simulink model "Neurofeedback_GetConnectivy_Validation"  (R2021b)
settings: Solver=VariableStepAuto  StartTime=0.0  StopTime=90  RelTol=1e-3
libraries: simrfV2util1 x6, simulink x3, simrfV2elements x2
settings Model: Creator=mariodelossantos  LastModifiedBy=mariodelossantos

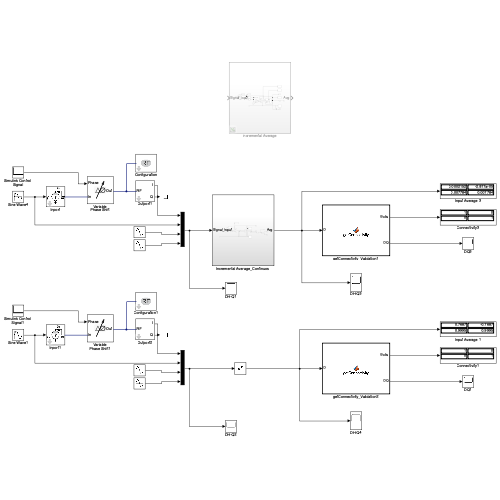
[thumbnail: Simulink's stored preview of the top-level diagram]
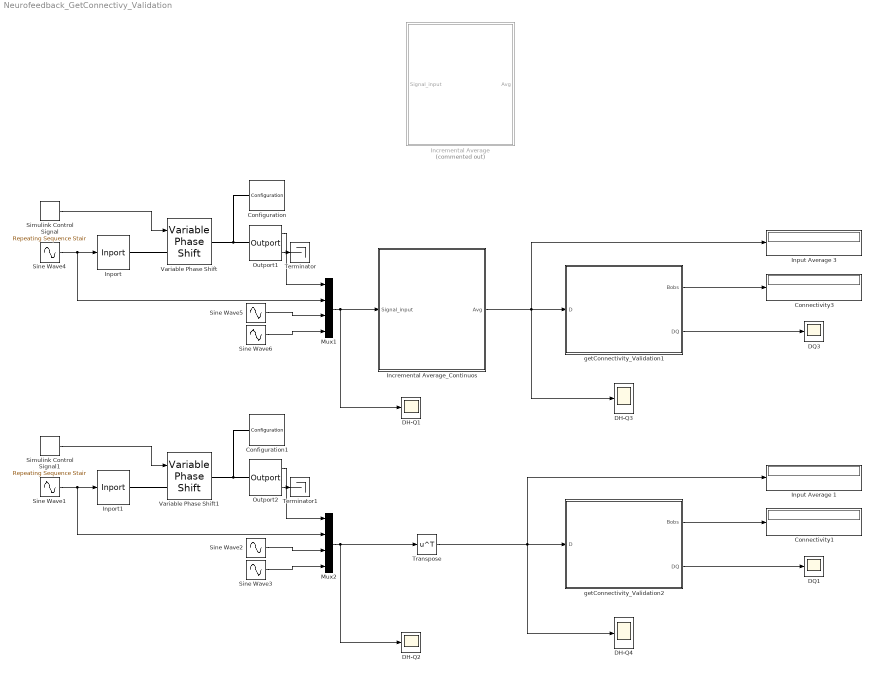
== system Neurofeedback_GetConnectivy_Validation ==
  Configuration : simrfV2util1/Configuration  AutoFreq=on  Tones=[1] GHz  Harmonics=[7]  NormalizeCarrierPower=on  SolverType=Auto  UseCCode=on  StepSize=1e-3/8 s  AddNoise=on  defaultRNG=on  Seed=0  Temperature=290.0 K  SolverDelFlag=0  AbsTol=1e-6  RelTol=1e-3  MaxIter=10  ErrorEstimationType=2-norm over all variables  EnableInterpFilter=off  HiddenFIRfilterControllerParam=on  SmallSignalApprox=off  AllSimFreqs=on  SimFreqs=[] Hz  SimFreqsInternal=[]  SamplesPerFrame=1
      settings: SourceProductBaseCode=RB
  Configuration1 : simrfV2util1/Configuration  AutoFreq=on  Tones=[1] GHz  Harmonics=[7]  NormalizeCarrierPower=on  SolverType=Auto  UseCCode=on  StepSize=1e-3/8 s  AddNoise=on  defaultRNG=on  Seed=0  Temperature=290.0 K  SolverDelFlag=0  AbsTol=1e-6  RelTol=1e-3  MaxIter=10  ErrorEstimationType=2-norm over all variables  EnableInterpFilter=off  HiddenFIRfilterControllerParam=on  SmallSignalApprox=off  AllSimFreqs=on  SimFreqs=[] Hz  SimFreqsInternal=[]  SamplesPerFrame=1
      settings: SourceProductBaseCode=RB
  Connectivity1 : Display
  Connectivity3 : Display
  DH-Q{1..4} (4 alike) : Scope
  DQ1 : Scope
  DQ3 : Scope
  Incremental Average : Subsystem  Commented=on
  "Incremental Average_Continuos " : Subsystem
  Inport : simrfV2util1/Inport  SimulinkInputSignalType=Power  CarrierFreq=1e9 Hz  ZS=50  InternalGrounding=on
      settings: SourceProductBaseCode=RB
  Inport1 : simrfV2util1/Inport  SimulinkInputSignalType=Power  CarrierFreq=1e9 Hz  ZS=50  InternalGrounding=on
      settings: SourceProductBaseCode=RB
  Input Average 1 : Display
  Input Average 3 : Display
  Mux1 : Mux
  Mux2 : Mux
  Outport1 : simrfV2util1/Outport  SensorType=Power  OutputFormat=In-phase and Quadrature Baseband  CarrierFreq=1e9 Hz  ZL=50  InternalGrounding=on  StepSize=1.25e-10 s  AutoStep=on
      settings: SourceProductBaseCode=RB
  Outport2 : simrfV2util1/Outport  SensorType=Power  OutputFormat=In-phase and Quadrature Baseband  CarrierFreq=1e9 Hz  ZL=50  InternalGrounding=on  StepSize=1.25e-10 s  AutoStep=on
      settings: SourceProductBaseCode=RB
  Simulink Control Signal : simulink/Sources/Repeating Sequence Stair  OutValues=180  tsamp=1e-3  OutMin=[]  OutMax=[]  OutDataTypeStr=double  OutputDataTypeScalingMode=double  OutDataType=fixdt(0,8)  ConRadixGroup=Best Precision: Vector-wise  OutScaling=2^-12
  Simulink Control Signal1 : simulink/Sources/Repeating Sequence Stair  OutValues=180  tsamp=1e-3  OutMin=[]  OutMax=[]  OutDataTypeStr=double  OutputDataTypeScalingMode=double  OutDataType=fixdt(0,8)  ConRadixGroup=Best Precision: Vector-wise  OutScaling=2^-12
  Sine Wave1 : Sin  Amplitude=1.2  SampleTime=0
  Sine Wave{2..3,5..6} (4 alike) : Sin  Frequency=1.4  SampleTime=0
  Sine Wave4 : Sin  Amplitude=1.2  SampleTime=0
  Terminator : Terminator
  Terminator1 : Terminator
  Transpose : Math  Operator=transpose  SaturateOnIntegerOverflow=on
  Variable Phase Shift : simrfV2elements/Variable Phase Shift  classname=varphase  PhaseShift_unit=deg  SparamZ0=50  InternalGrounding=on
      settings: SourceProductBaseCode=RB
  Variable Phase Shift1 : simrfV2elements/Variable Phase Shift  classname=varphase  PhaseShift_unit=deg  SparamZ0=50  InternalGrounding=on
      settings: SourceProductBaseCode=RB
  getConnectivity_Validation1 : MATLAB Function  TreatAsAtomicUnit=on  SystemSampleTime=0
  getConnectivity_Validation2 : MATLAB Function  TreatAsAtomicUnit=on  SystemSampleTime=0
  wires:
  getConnectivity_Validation1/1(Bobs) -> Connectivity3/1
  getConnectivity_Validation1/2(DQ) -> DQ3/1
  Sine Wave4/1 -> Mux1/2, Inport/1
  Simulink Control Signal/1 -> Variable Phase Shift/1
  Outport1/2 -> Terminator/1
  Sine Wave6/1 -> Mux1/4
  Sine Wave5/1 -> Mux1/3
  Mux1/1 -> "Incremental Average_Continuos "/1(Signal_input), DH-Q1/1
  getConnectivity_Validation2/1(Bobs) -> Connectivity1/1
  Sine Wave1/1 -> Mux2/2, Inport1/1
  Sine Wave3/1 -> Mux2/4
  Mux2/1 -> Transpose/1, DH-Q2/1
  getConnectivity_Validation2/2(DQ) -> DQ1/1
  Transpose/1 -> DH-Q4/1, getConnectivity_Validation2/1("D "), Input Average 1/1
  Outport2/2 -> Terminator1/1
  Sine Wave2/1 -> Mux2/3
  Simulink Control Signal1/1 -> Variable Phase Shift1/1
  "Incremental Average_Continuos "/1(Avg) -> DH-Q3/1, Input Average 3/1, getConnectivity_Validation1/1("D ")
  Outport1/1 -> Mux1/1
  Outport2/1 -> Mux2/1
  connections:
  Variable Phase Shift/RConn1 -- Configuration/LConn1 -- Outport1/LConn1
  Inport/RConn1 -- Variable Phase Shift/LConn1
  Outport2/LConn1 -- Variable Phase Shift1/RConn1 -- Configuration1/LConn1
  Inport1/RConn1 -- Variable Phase Shift1/LConn1

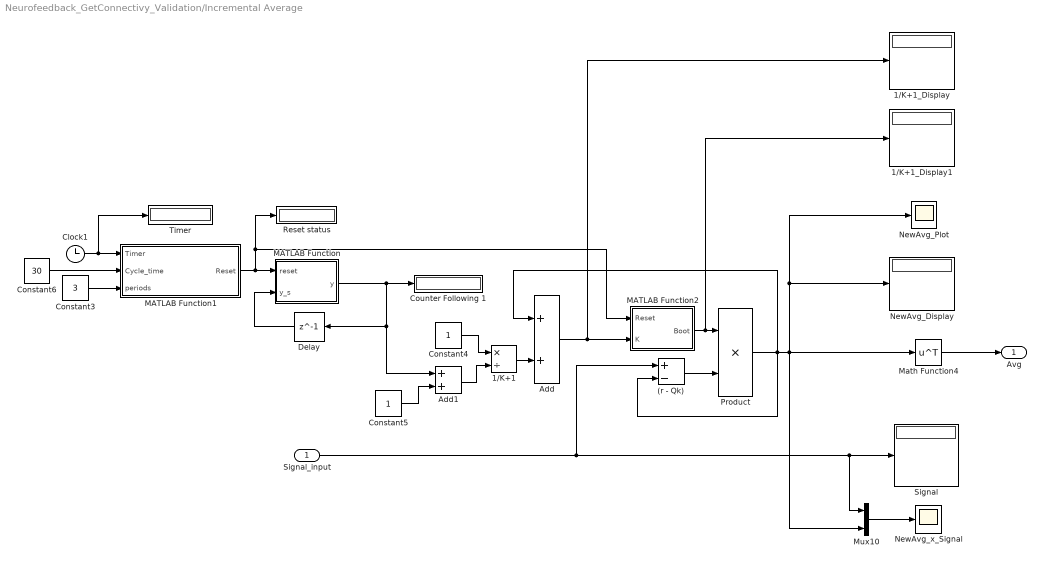
== system Neurofeedback_GetConnectivy_Validation/Incremental Average ==
  Signal_input : Inport
  (r - Qk) : Sum  Inputs=+-
  1/K+1 : Product  Inputs=*/
  1/K+1_Display : Display
  1/K+1_Display1 : Display
  Add : Sum
  Add1 : Sum
  Clock1 : Clock
  Constant3 : Constant  Value=3
  Constant4 : Constant
  Constant5 : Constant
  Constant6 : Constant  Value=30
  Counter Following 1 : Display
  Delay : Delay  DelayLength=1  InitialCondition=0
  MATLAB Function : MATLAB Function  TreatAsAtomicUnit=on
  MATLAB Function1 : MATLAB Function  TreatAsAtomicUnit=on
  MATLAB Function2 : MATLAB Function  TreatAsAtomicUnit=on
  Math Function4 : Math  Operator=transpose  SaturateOnIntegerOverflow=on
  Mux10 : Mux  Inputs=2
  NewAvg_Display : Display
  NewAvg_Plot : Scope
  NewAvg_x_Signal : Scope
  Product : Product
  Reset status : Display
  Signal : Display
  Timer : Display
  Avg : Outport
  wires:
  (r - Qk)/1 -> Product/2
  Signal_input/1 -> Mux10/1, Signal/1, (r - Qk)/1
  Add/1 -> 1/K+1_Display/1, MATLAB Function2/2(K)
  Mux10/1 -> NewAvg_x_Signal/1
  Product/1 -> Add/1, (r - Qk)/2, Mux10/2, NewAvg_Plot/1, NewAvg_Display/1, Math Function4/1
  Math Function4/1 -> Avg/1
  Constant4/1 -> 1/K+1/1
  Constant5/1 -> Add1/2
  Add1/1 -> 1/K+1/2
  1/K+1/1 -> Add/2
  MATLAB Function/1(y) -> Delay/1, Add1/1, Counter Following 1/1
  Delay/1 -> MATLAB Function/2(y_s)
  MATLAB Function1/1(Reset) -> Reset status/1, MATLAB Function2/1(Reset), MATLAB Function/1(reset)
  Constant6/1 -> MATLAB Function1/2(Cycle_time)
  Constant3/1 -> MATLAB Function1/3(periods)
  Clock1/1 -> MATLAB Function1/1(Timer), Timer/1
  MATLAB Function2/1(Boot) -> 1/K+1_Display1/1, Product/1

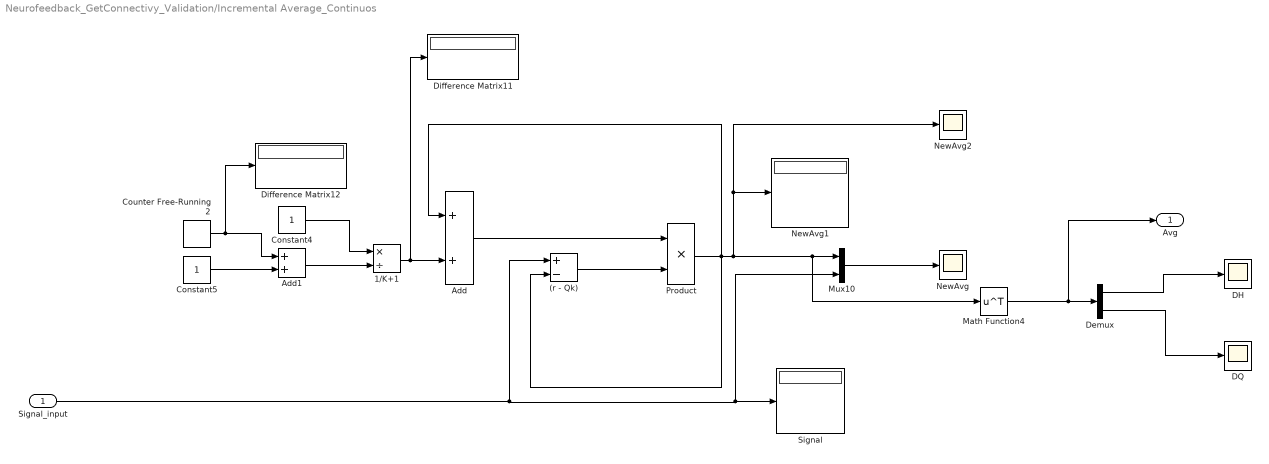
== system Neurofeedback_GetConnectivy_Validation/Incremental Average_Continuos  ==
  Signal_input : Inport
  (r - Qk) : Sum  Inputs=+-
  1/K+1 : Product  Inputs=*/
  Add : Sum
  Add1 : Sum
  Constant4 : Constant
  Constant5 : Constant
  Counter Free-Running2 : simulink/Sources/Counter Free-Running  NumBits=16  tsamp=-1
  DH : Scope
  DQ : Scope
  Demux : Demux  Outputs=2
  Difference Matrix11 : Display
  Difference Matrix12 : Display
  Math Function4 : Math  Operator=transpose  SaturateOnIntegerOverflow=on
  Mux10 : Mux  Inputs=2
  NewAvg : Scope
  NewAvg1 : Display
  NewAvg2 : Scope
  Product : Product
  Signal : Display
  Avg : Outport
  wires:
  1/K+1/1 -> Difference Matrix11/1, Add/2
  Counter Free-Running2/1 -> Difference Matrix12/1, Add1/1
  (r - Qk)/1 -> Product/2
  Signal_input/1 -> Signal/1, Mux10/2, (r - Qk)/1
  Add/1 -> Product/1
  Mux10/1 -> NewAvg/1
  Product/1 -> Add/1, (r - Qk)/2, NewAvg2/1, NewAvg1/1, Math Function4/1, Mux10/1
  Add1/1 -> 1/K+1/2
  Constant5/1 -> Add1/2
  Constant4/1 -> 1/K+1/1
  Math Function4/1 -> Avg/1, Demux/1
  Demux/2 -> DQ/1
  Demux/1 -> DH/1

== matlab function Neurofeedback_GetConnectivy_Validation/Incremental Average/MATLAB Function ==
  data: reset input; y_s input; y output
function y = fcn(reset, y_s)

if reset == 1
    y = 0;
else 
    y = y_s + 1;
end

== matlab function Neurofeedback_GetConnectivy_Validation/Incremental Average/MATLAB Function1 ==
  data: Timer input; Reset output; Cycle_time input; periods input
function Reset  = fcn(Timer, Cycle_time, periods)

temp = 0;
PCycles = zeros(periods,1);
for i = 1:periods
    PCycles(i) = i * Cycle_time;
    if (Timer >= PCycles(i) && Timer <= PCycles(i)+1)
        temp = 1;
        break
    else
        temp = 0;
    end
end 
Reset = temp;

== matlab function Neurofeedback_GetConnectivy_Validation/getConnectivity_Validation2 ==
  data: D input; Bobs output; DQ output
function [Bobs,DQ]  = getConnectivity(D)

    DQ = zeros(1, 2);
    DQ(1,1)=D(1,1);
    DQ(1,2)=D(1,2);


    DH = zeros(1,2);
    DH(1,1)=D(1,3);
    DH(1,2)=D(1,4);

    rThresh= 0.6; % [0..1] A threshold on the correlation.

    [nSamples, nChannels, nHb]=size(DQ);

    C = nan(nChannels, nChannels, nHb); %Matrix of channel pairwise correlations;

    %This part of the algorithm is HIGHLY inefficient but it does the job for now
    %but might not be sufficiently fast for "real time" neurofeedback

    for iHb = 1:nHb
        for iCh=1:nChannels
            for jCh=iCh:nChannels

                if iCh == jCh

                 C(iCh,jCh,iHb) = 1;

               else

                 C(iCh,jCh,iHb) = xcorr2(DQ(:,iCh,iHb),DQ(:,jCh,iHb));

                end
            end

        end

    end

    %Threshold/Binarize C


    tmp = C > rThresh;

    %Finally "merge" accross Hb species

    Bobs = all(tmp,3); %Apply the AND function across Hb species.

== matlab function Neurofeedback_GetConnectivy_Validation/Incremental Average/MATLAB Function2 ==
  data: Reset input; K input; Boot output
function Boot = fcn(Reset, K)

    temp = ones(4, 1);
    Boot = [0;0;0;0];
    if Reset == 1
        temp = Boot;
    else 
        temp = K;
    end 

    Boot = temp;

== matlab function Neurofeedback_GetConnectivy_Validation/getConnectivity_Validation1 ==
  data: D input; Bobs output; DQ output
function [Bobs,DQ]  = getConnectivity(D)

    DQ = zeros(1, 2);
    DQ(1,1)=D(1,1);
    DQ(1,2)=D(1,2);


    DH = zeros(1,2);
    DH(1,1)=D(1,3);
    DH(1,2)=D(1,4);

    rThresh= 0.6; % [0..1] A threshold on the correlation.

    [nSamples, nChannels, nHb]=size(DQ);

    C = nan(nChannels, nChannels, nHb); %Matrix of channel pairwise correlations;

    %This part of the algorithm is HIGHLY inefficient but it does the job for now
    %but might not be sufficiently fast for "real time" neurofeedback

    for iHb = 1:nHb
        for iCh=1:nChannels
            for jCh=iCh:nChannels

                if iCh == jCh

                 C(iCh,jCh,iHb) = 1;

               else

                 C(iCh,jCh,iHb) = xcorr2(DQ(:,iCh,iHb),DQ(:,jCh,iHb));

                end
            end

        end

    end

    %Threshold/Binarize C


    tmp = C > rThresh;

    %Finally "merge" accross Hb species

    Bobs = all(tmp,3); %Apply the AND function across Hb species.
